simulink model "plane_model_2"  (R2020b)
settings: Solver=VariableStepAuto  StartTime=0.0  StopTime=80  RelTol=1e-3
values from neighbouring files (symbols this model uses):
  A = [-1.064 1; 290.26 0]    [parameters.m]
  B = [-0.25; -331.4]    [parameters.m]
  C = [-123.34 0; 0 1]    [parameters.m]
  D = [-13.51; 0]    [parameters.m]
  dT1 = 0.75    [parameters.m]
  dT2 = 0.25    [parameters.m]
  ELEV_INIT = 10000    [parameters.m]
  ELEV_TARGET = 795    [parameters.m]
  LAT_INIT = 34.2329    [parameters.m]
  LAT_OBS = 34.61916    [parameters.m]
  LAT_TARGET = 34.6588    [parameters.m]
  LON_INIT = -119.4573    [parameters.m]
  LON_OBS = -118.8429    [parameters.m]
  LON_TARGET = -118.769745    [parameters.m]
  Vel = 1021.08    [parameters.m]
undefined symbols (not defined in the file or in its folder): Earth, K, L, WGS84
libraries: simulink x3, aerolibfltsims x2, pid_lib x1, aerolibtransform2 x1
settings Model: Creator=Markus  LastModifiedBy=Markus

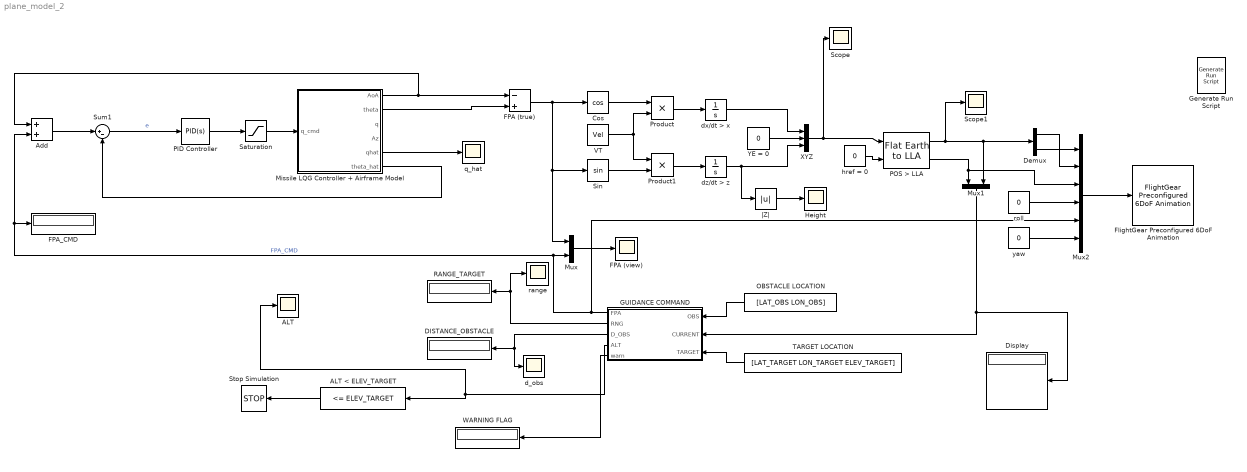
== system plane_model_2 ==
  ALT : Scope
  ALT < ELEV_TARGET : simulink/Logic and Bit Operations/Compare To Constant  relop=<=  const=ELEV_TARGET  OutDataTypeStr=boolean
  Add : Sum
  Cos : Trigonometry  Operator=cos
  DISTANCE_OBSTACLE : Display
  Demux : Demux  Outputs=2
  Display : Display
  FPA (true) : Sum  Inputs=-+
  FPA (view) : Scope
  FPA_CMD : Display
  FlightGear Preconfigured 6DoF Animation : aerolibfltsims/FlightGear Preconfigured 6DoF Animation  xFlightGearVersion=v2019.1  DestinationIpAddress=127.0.0.1  DestinationPort=5502  SampleTime=1/30  packetVersion=24
  GUIDANCE COMMAND : MATLAB Function  TreatAsAtomicUnit=on
  Generate Run Script : aerolibfltsims/Generate Run Script  Architecture=Win64  dataFlow=Send  GeometryModelName=c172p  AirportId=KSFO  RunwayId=10L  InitialAltitude=7224  InitialHeading=113  OffsetDistance=4.72  OffsetAzimuth=0  InstallScenery=off  DisableShaders=on  OriginAddress=127.0.0.1  DestinationPort=5502  OriginPort=5505  LocalAddress=127.0.0.1  OutputFileName=runfg_model_2.bat  FlightGearBaseDirectory=C:\Program Files\FlightGear 2020.1.3
  Height : Scope
  Missile LQG Controller + Airframe Model : Subsystem
  Mux : Mux  Inputs=2
  Mux1 : Mux  Inputs=2
  Mux2 : Mux  Inputs=6
  OBSTACLE LOCATION : Constant  Value=[LAT_OBS LON_OBS]
  PID Controller : pid_lib/PID Controller  Controller=PID  Form=Parallel  TimeDomain=Continuous-time  UseExternalTs=off  SampleTime=-1  IntegratorMethod=Forward Euler  FilterMethod=Forward Euler  ControllerParametersSource=internal  P=-1  I=0  D=0  UseFilter=on  N=100  TunerSelectOption=Transfer Function Based (PID Tuner App)  InitialConditionSource=internal  InitialConditionForIntegrator=0  InitialConditionForFilter=0  DifferentiatorICPrevScaledInput=0  ExternalReset=none  TrackingMode=off  Kt=1  LimitOutput=off  SatLimitsSource=internal  UpperSaturationLimit=inf  LowerSaturationLimit=-inf  LinearizeAsGain=on  AntiWindupMode=none  Kb=1  POutMin=[]  POutMax=[]  IOutMin=[]  IOutMax=[]  DOutMin=[]  DOutMax=[]  NOutMin=[]  NOutMax=[]  SumOutMin=[]  SumOutMax=[]  SaturationOutMin=[]  SaturationOutMax=[]  PParamMin=[]  PParamMax=[]  IParamMin=[]  IParamMax=[]  DParamMin=[]  DParamMax=[]  NParamMin=[]  NParamMax=[]  KbParamMin=[]  KbParamMax=[]  KtParamMin=[]  KtParamMax=[]  KbOutMin=[]  KbOutMax=[]  KtOutMin=[]  KtOutMax=[]  IntegratorOutMin=[]  IntegratorOutMax=[]  FilterOutMin=[]  FilterOutMax=[]  SumI1OutMin=[]  SumI1OutMax=[]  SumI2OutMin=[]  SumI2OutMax=[]  SumI3OutMin=[]  SumI3OutMax=[]  SumI4OutMin=[]  SumI4OutMax=[]  SumDOutMin=[]  SumDOutMax=[]  DifferentiatorOutMin=[]  DifferentiatorOutMax=[]  FilterDiffOutCoefMin=[]  FilterDiffOutCoefMax=[]  ReciprocalOutMin=[]  ReciprocalOutMax=[]  SumDenOutMin=[]  SumDenOutMax=[]  SumNumOutMin=[]  SumNumOutMax=[]  DivideOutMin=[]  DivideOutMax=[]  UdiffTsProdOutMin=[]  UdiffTsProdOutMax=[]  NTsProdOutMin=[]  NTsProdOutMax=[]  UintegralTsProdOutMin=[]  UintegralTsProdOutMax=[]  UngainTsProdOutMin=[]  UngainTsProdOutMax=[]  IntegratorContinuousStateAttributes=''  IntegratorStateMustResolveToSignalObject=off  IntegratorRTWStateStorageClass=Auto  FilterContinuousStateAttributes=''  FilterStateMustResolveToSignalObject=off  FilterRTWStateStorageClass=Auto  ParallelPVariant=InternalParameters  IdealPVariant=Disabled  IVariant=InternalParameters  DVariant=InternalParameters  IntegratorVariant=Continuous  SatVariant=Disabled  AWVariant=Passthrough  PCopyVariant=Disabled  TRVariant=Disabled  FdbkBlocksVariant=Forward  IdealPFdbkVariant=Disabled  SatFdbkVariant=Disabled  DerivativeFilterVariant=ContFilter  NVariant=InternalParameters  NCopyVariant=Disabled  FilterICVariant=InternalICsFilter  IntegratorICVariant=InternalICs  ExternalResetVariant=Disabled  TRSumVariant=Passthrough  SumFdbkVariant=Disabled  SumVariant=Sum_PID  TsampFilterVariant=InternalTs  TsampNgainVariant=Passthrough  TsampIntegralVariant=Passthrough  ExternalSaturationOutDataTypeStr=Inherit: Same as second input
  POS > LLA : aerolibtransform2/Flat Earth to LLA  units=Metric (MKS)  ptype=Earth (WGS84)  F=1/298.257223563  R=6378137  refPosPort=off  LL0=[LAT_INIT LON_INIT]  psi=yaw_init
  Product : Product
  Product1 : Product
  RANGE_TARGET : Display
  Saturation : Saturate
  Scope : Scope
  Scope1 : Scope
  Sin : Trigonometry
  Stop Simulation : Stop
  Sum1 : Sum  Inputs=|+-
  TARGET LOCATION : Constant  Value=[LAT_TARGET LON_TARGET ELEV_TARGET]
  VT : Constant  Value=Vel
  WARNING FLAG : Display
  XYZ : Mux  Inputs=3
  YE = 0 : Constant  Value=0
  d_obs : Scope
  dx/dt > x : Integrator
  dz/dt > z : Integrator  InitialCondition=-ELEV_INIT
  href = 0 : Constant  Value=0
  q_hat : Scope
  range : Scope
  roll : Constant  Value=0
  yaw : Constant  Value=0
  |Z| : Abs
  wires:
  Saturation/1 -> Missile LQG Controller + Airframe Model/1(q_cmd)
  Missile LQG Controller + Airframe Model/1(AoA) -> Add/1, FPA (true)/1
  Missile LQG Controller + Airframe Model/2(theta) -> FPA (true)/2
  Missile LQG Controller + Airframe Model/6(theta_hat) -> Sum1/2
  PID Controller/1 -> Saturation/1
  Sum1/1 -> PID Controller/1  "e"
  Add/1 -> Sum1/1
  GUIDANCE COMMAND/1(FPA) -> FPA_CMD/1, Add/2, Mux/2, Mux2/5  "FPA_CMD"
  FPA (true)/1 -> Cos/1, Sin/1, Mux/1
  Mux/1 -> FPA (view)/1
  Cos/1 -> Product/1
  Sin/1 -> Product1/2
  VT/1 -> Product/2, Product1/1
  Product/1 -> dx/dt > x/1
  Product1/1 -> dz/dt > z/1
  YE = 0/1 -> XYZ/2
  dz/dt > z/1 -> |Z|/1, XYZ/3
  dx/dt > x/1 -> XYZ/1
  |Z|/1 -> Height/1
  Missile LQG Controller + Airframe Model/5(qhat) -> q_hat/1
  XYZ/1 -> Scope/1, POS > LLA/1
  href = 0/1 -> POS > LLA/2
  POS > LLA/2 -> Mux2/3, Mux1/1
  POS > LLA/1 -> Scope1/1, Demux/1, Mux1/2
  OBSTACLE LOCATION/1 -> GUIDANCE COMMAND/1(OBS)
  TARGET LOCATION/1 -> GUIDANCE COMMAND/3(TARGET)
  Mux1/1 -> Display/1, GUIDANCE COMMAND/2(CURRENT)
  GUIDANCE COMMAND/2(RNG) -> range/1, RANGE_TARGET/1
  GUIDANCE COMMAND/3(D_OBS) -> d_obs/1, DISTANCE_OBSTACLE/1
  GUIDANCE COMMAND/5(warn) -> WARNING FLAG/1
  GUIDANCE COMMAND/4(ALT) -> ALT < ELEV_TARGET/1, ALT/1
  ALT < ELEV_TARGET/1 -> Stop Simulation/1
  Demux/1 -> Mux2/2
  Demux/2 -> Mux2/1
  roll/1 -> Mux2/4
  yaw/1 -> Mux2/6
  Mux2/1 -> FlightGear Preconfigured 6DoF Animation/1

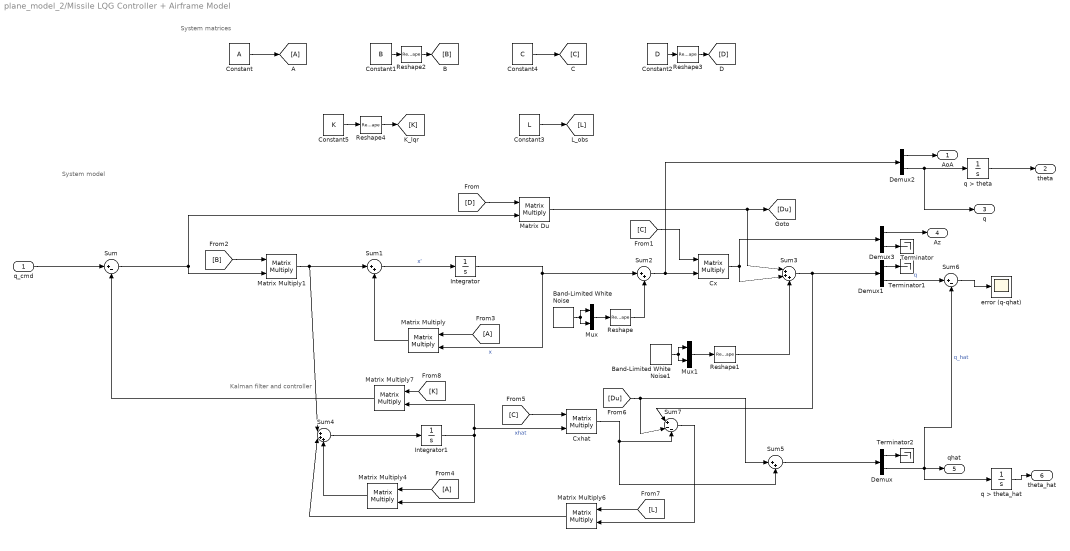
== system plane_model_2/Missile LQG Controller + Airframe Model ==
  note: System model
  note: Kalman filter and controller
  note: System matrices
  q_cmd : Inport
  Band-Limited White Noise : simulink/Sources/Band-Limited White Noise  Cov=[0.00000001]  Ts=dT1  seed=[23341]
  Band-Limited White Noise1 : simulink/Sources/Band-Limited White Noise  Cov=[0.00001]  Ts=dT2  seed=[23341]
  Constant : Constant  Value=A
  Constant1 : Constant  Value=B
  Constant2 : Constant  Value=D
  Constant3 : Constant  Value=L
  Constant4 : Constant  Value=C
  Constant5 : Constant  Value=K
  Cx : Product  Multiplication=Matrix(*)
  Cxhat : Product  Multiplication=Matrix(*)
  Demux{,1..3} (4 alike) : Demux  Outputs=2
  Integrator : Integrator
  Integrator1 : Integrator
  Matrix Du : Product  Multiplication=Matrix(*)
  Matrix Multiply{,1,4,6..7} (5 alike) : Product  Multiplication=Matrix(*)
  Mux : Mux  Inputs=2
  Mux1 : Mux  Inputs=2
  Reshape{,1..3} (4 alike) : Reshape  OutputDimensionality=Customize  OutputDimensions=[2,1]
  Reshape4 : Reshape  OutputDimensionality=Customize  OutputDimensions=[1,2]
  Sum : Sum  Inputs=|+-
  Sum1 : Sum  Inputs=|++
  Sum2 : Sum  Inputs=|++
  Sum3 : Sum  Inputs=|+++
  Sum4 : Sum  Inputs=|+++
  Sum5 : Sum  Inputs=|++
  Sum6 : Sum  Inputs=|+-
  Sum7 : Sum  Inputs=|+--
  Terminator : Terminator
  Terminator1 : Terminator
  Terminator2 : Terminator
  error (q-qhat) : Scope
  q > theta : Integrator
  q > theta_hat : Integrator
  AoA : Outport
  theta : Outport  Port=2
  q : Outport  Port=3
  Az : Outport  Port=4
  qhat : Outport  Port=5
  theta_hat : Outport  Port=6
  wires:
  Cxhat/1 -> Sum7/3, Sum5/2
  Demux/2 -> qhat/1, q > theta_hat/1, Sum6/2  "q_hat"
  Matrix Multiply7/1 -> Sum/2
  Band-Limited White Noise/1 -> Mux/1, Mux/2
  [D] -> Matrix Du/1
  Sum5/1 -> Demux/1
  Matrix Multiply1/1 -> Sum1/1, Sum4/1
  Sum2/1 -> Demux2/1, Cx/2
  Demux1/1 -> Terminator1/1
  Integrator1/1 -> Matrix Multiply7/2, Cxhat/2, Matrix Multiply4/2  "xhat"
  [Du] -> Sum7/2, Sum5/1
  Integrator/1 -> Matrix Multiply/2, Sum2/1  "x"
  Constant/1 -> [A]
  Constant5/1 -> Reshape4/1
  Constant3/1 -> [L]
  Mux/1 -> Reshape/1
  Matrix Multiply/1 -> Sum1/2
  Demux2/2 -> q/1, q > theta/1
  [C] -> Cx/1
  q > theta/1 -> theta/1
  [A] -> Matrix Multiply4/1
  Sum3/1 -> Sum7/1, Demux1/1
  Sum6/1 -> error (q-qhat)/1
  [L] -> Matrix Multiply6/1
  Sum/1 -> Matrix Multiply1/2, Matrix Du/2
  Mux1/1 -> Reshape1/1
  Constant2/1 -> Reshape3/1
  Constant4/1 -> [C]
  [C] -> Cxhat/1
  Reshape/1 -> Sum2/2
  [B] -> Matrix Multiply1/1
  Demux3/1 -> Az/1
  Demux1/2 -> Sum6/1  "q"
  Demux2/1 -> AoA/1
  Matrix Multiply4/1 -> Sum4/3
  Reshape3/1 -> [D]
  Matrix Multiply6/1 -> Sum4/2
  Sum1/1 -> Integrator/1  "x'"
  Matrix Du/1 -> Sum3/1, [Du]
  Cx/1 -> Demux3/1, Sum3/2
  Sum4/1 -> Integrator1/1
  Demux3/2 -> Terminator/1
  [A] -> Matrix Multiply/1
  q > theta_hat/1 -> theta_hat/1
  Reshape1/1 -> Sum3/3
  q_cmd/1 -> Sum/1
  Band-Limited White Noise1/1 -> Mux1/1, Mux1/2
  Reshape2/1 -> [B]
  Demux/1 -> Terminator2/1
  Sum7/1 -> Matrix Multiply6/2
  Constant1/1 -> Reshape2/1
  Reshape4/1 -> [K]
  [K] -> Matrix Multiply7/1

== matlab function plane_model_2/GUIDANCE COMMAND ==
  data: OBS input; FPA output; CURRENT input; TARGET input; RNG output; D_OBS output; ALT output; warn output
function [FPA, RNG, D_OBS, ALT, warn] = fcn(OBS, CURRENT, TARGET)
    
R = 6371e3;
d2r = pi/180;

%OBSTACLE LOCATION
LAT_OBS = OBS(1);
LON_OBS = OBS(2);

%OBSTACLE TRESHOLD (ZONE)
thresh = 2000;

%TARGET LOCATION
LAT_TARGET = TARGET(1);
LON_TARGET = TARGET(2);
ELEV_TARGET = TARGET(3);

%CURRENT LOCATION
ELEV_CUR = CURRENT(1);
LAT_CUR = CURRENT(2);
LON_CUR = CURRENT(3);

%% distance to target
l1 = LAT_CUR*d2r;
u1 = LON_CUR*d2r;
l2 = LAT_TARGET*d2r;
u2 = LON_TARGET*d2r;
dh = abs(ELEV_TARGET-ELEV_CUR);

dl = l2 - l1;
du = u2 - u1;

% haversine formular 
a = sin(dl/2)^2 + cos(l1)*cos(l2)*sin(du/2)^2;
c = 2*atan2(sqrt(a),sqrt(1-a));
d = R*c;

%% distance from the obstacle
l3 = LAT_OBS*d2r;
u3 = LON_OBS*d2r;

dl_2 = l3 - l1;
du_2 = u3 - u1;

a_2 = sin(dl_2/2)^2 + cos(l1)*cos(l2)*sin(du_2/2)^2;
c_2 = 2*atan2(sqrt(a_2),sqrt(1-a_2));
d_obs = R*c_2;

%% current range (from target)-range > distance
range = sqrt(d^2+dh^2);

%% calculate commanded flight path setpoint based on d_obs, range
if abs(d_obs) >= thresh
    w = 0;
    FPA_CMD = atan(dh/d);
else
    w = 1;
    FPA_CMD = 0;
end

%% output variables
FPA = FPA_CMD;
RNG = range;
D_OBS = d_obs;
warn = w;
ALT = ELEV_CUR;
